simulink model "que4"  (R2020a)
settings: Solver=VariableStepAuto  StartTime=0.0  StopTime=10.0  RelTol=1e-3
libraries: simulink x1
settings Model: Creator=kiran  LastModifiedBy=kiran

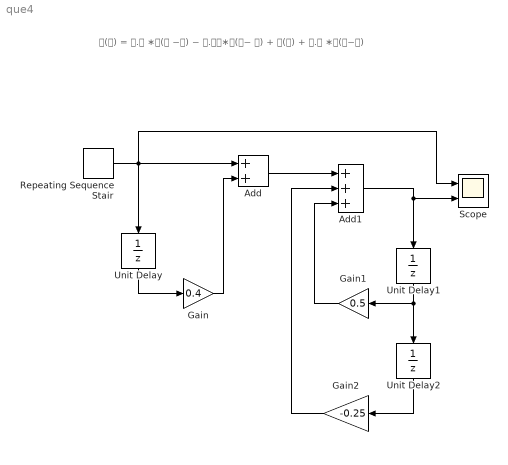
== system que4 ==
  note: 𝐲(𝐧) = 𝟎.𝟓 ∗𝐲(𝐧 −𝟏) − 𝟎.𝟐𝟓∗𝐲(𝐧− 𝟐) + 𝐱(𝐧) + 𝟎.𝟒 ∗𝐱(𝐧−𝟏)
  Add : Sum
  Add1 : Sum  Inputs=+++
  Gain : Gain  Gain=0.4
  Gain1 : Gain  Gain=0.5
  Gain2 : Gain  Gain=-0.25
  Repeating Sequence Stair : simulink/Sources/Repeating Sequence Stair  OutValues=[1 0 0 0 0].'  tsamp=-1  OutMin=[]  OutMax=[]  OutDataTypeStr=double  OutputDataTypeScalingMode=double  OutDataType=fixdt(0,8)  ConRadixGroup=Best Precision: Vector-wise  OutScaling=2^-12
  Scope : Scope  NumInputPorts=2
  Unit Delay : UnitDelay  SampleTime=-1  HasFrameUpgradeWarning=on
  Unit Delay1 : UnitDelay  SampleTime=-1  HasFrameUpgradeWarning=on
  Unit Delay2 : UnitDelay  SampleTime=-1  HasFrameUpgradeWarning=on
  wires:
  Repeating Sequence Stair/1 -> Scope/1, Unit Delay/1, Add/1
  Unit Delay/1 -> Gain/1
  Gain/1 -> Add/2
  Add/1 -> Add1/1
  Add1/1 -> Scope/2, Unit Delay1/1
  Unit Delay1/1 -> Gain1/1, Unit Delay2/1
  Gain1/1 -> Add1/3
  Unit Delay2/1 -> Gain2/1
  Gain2/1 -> Add1/2
